simulink model "lab4_2"  (R2016b)
settings: Solver=VariableStepAuto  StartTime=0.0  StopTime=totaltime  RelTol=1e-3
undefined symbols (not defined in the file or in its folder): h
libraries: xbsIndex_r4 x1157
(part 1 of 4)
settings Model: Creator=rm101  LastModifiedBy=rm101

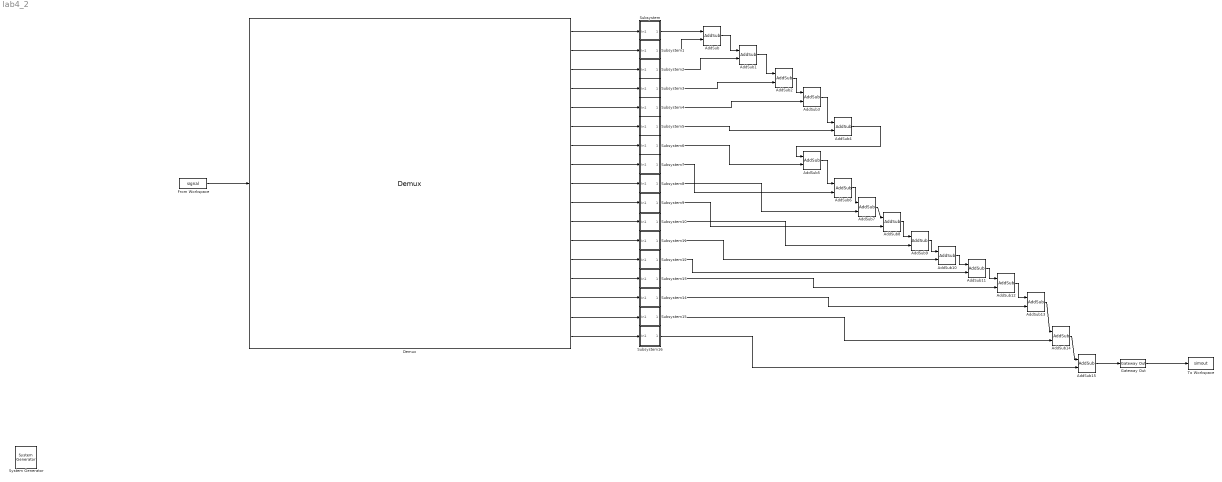
== system lab4_2 ==
  " System Generator" : xbsIndex_r4/ System Generator  Tag=genX  xilinxfamily=zynq  part=xc7z020  speed=-1  package=clg484  synthesis_tool=Vivado  clock_wrapper=Clock Enables  directory=C:/Users/rm101/lab4  proj_type=Vivado  Synth_file=Vivado Synthesis Defaults  Impl_file=Vivado Implementation Defaults  testbench=off  simulink_period=st  sysclk_period=10  dcm_input_clock_period=10  incr_netlist=off  trim_vbits=Everywhere in SubSystem  dbl_ovrd=According to Block Masks  core_generation=According to Block Masks  run_coregen=off  deprecated_control=off  eval_field=0  block_type=sysgen
  AddSub{,1..15} (16 alike) : xbsIndex_r4/AddSub  mode=Addition  use_carryin=off  use_carryout=off  en=off  latency=0  precision=Full  arith_type=Unsigned  n_bits=16  bin_pt=14  quantization=Truncate  overflow=Wrap  use_behavioral_HDL=off  hw_selection=Fabric  pipelined=off  dbl_ovrd=off  block_type=addsub
  Demux : Demux  Outputs=17
  From Workspace : FromWorkspace  VariableName=signal  SampleTime=0
  Gateway Out : xbsIndex_r4/Gateway Out  inherit_from_input=off  hdl_port=on  rows=1  columns=1  UseAsDAC=off  DACChannel='1'  interface=None  automatic_assignment=on  address_offset=hex2dec('00')  intf_name=''  intf_description=''  timing_constraint=None  locs_specified=off  LOCs={}  io_standard={}  block_type=gatewayout
  Subsystem : Subsystem
  Subsystem1 : Subsystem
  Subsystem10 : Subsystem
  Subsystem11 : Subsystem
  Subsystem12 : Subsystem
  Subsystem13 : Subsystem
  Subsystem14 : Subsystem
  Subsystem15 : Subsystem
  Subsystem16 : Subsystem
  Subsystem2 : Subsystem
  Subsystem3 : Subsystem
  Subsystem4 : Subsystem
  Subsystem5 : Subsystem
  Subsystem6 : Subsystem
  Subsystem7 : Subsystem
  Subsystem8 : Subsystem
  Subsystem9 : Subsystem
  To Workspace : ToWorkspace  VariableName=simout  SaveFormat=Timeseries  SampleTime=-1
  wires:
  From Workspace/1 -> Demux/1
  Demux/1 -> Subsystem/1(In1)
  Demux/2 -> Subsystem1/1(In1)
  Demux/3 -> Subsystem2/1(In1)
  Demux/4 -> Subsystem3/1(In1)
  Demux/5 -> Subsystem4/1(In1)
  Demux/6 -> Subsystem5/1(In1)
  Demux/7 -> Subsystem6/1(In1)
  Demux/8 -> Subsystem7/1(In1)
  Demux/9 -> Subsystem8/1(In1)
  Demux/10 -> Subsystem9/1(In1)
  Demux/11 -> Subsystem10/1(In1)
  Demux/12 -> Subsystem11/1(In1)
  Demux/13 -> Subsystem12/1(In1)
  Demux/14 -> Subsystem13/1(In1)
  Demux/15 -> Subsystem14/1(In1)
  Demux/16 -> Subsystem15/1(In1)
  Demux/17 -> Subsystem16/1(In1)
  Subsystem/1(Out1) -> AddSub/1
  Subsystem1/1(Out1) -> AddSub/2
  AddSub/1 -> AddSub1/1
  Subsystem2/1(Out1) -> AddSub1/2
  AddSub1/1 -> AddSub2/1
  Subsystem3/1(Out1) -> AddSub2/2
  AddSub2/1 -> AddSub3/1
  Subsystem4/1(Out1) -> AddSub3/2
  AddSub3/1 -> AddSub4/1
  Subsystem5/1(Out1) -> AddSub4/2
  Subsystem6/1(Out1) -> AddSub5/2
  Subsystem7/1(Out1) -> AddSub6/2
  AddSub5/1 -> AddSub6/1
  AddSub6/1 -> AddSub7/1
  AddSub7/1 -> AddSub8/1
  AddSub8/1 -> AddSub9/1
  AddSub9/1 -> AddSub10/1
  AddSub10/1 -> AddSub11/1
  AddSub11/1 -> AddSub12/1
  AddSub12/1 -> AddSub13/1
  AddSub13/1 -> AddSub14/1
  AddSub4/1 -> AddSub5/1
  Gateway Out/1 -> To Workspace/1
  Subsystem8/1(Out1) -> AddSub7/2
  Subsystem9/1(Out1) -> AddSub8/2
  Subsystem10/1(Out1) -> AddSub9/2
  Subsystem11/1(Out1) -> AddSub10/2
  Subsystem12/1(Out1) -> AddSub11/2
  Subsystem13/1(Out1) -> AddSub12/2
  Subsystem14/1(Out1) -> AddSub13/2
  Subsystem15/1(Out1) -> AddSub14/2
  AddSub15/1 -> Gateway Out/1
  AddSub14/1 -> AddSub15/1
  Subsystem16/1(Out1) -> AddSub15/2

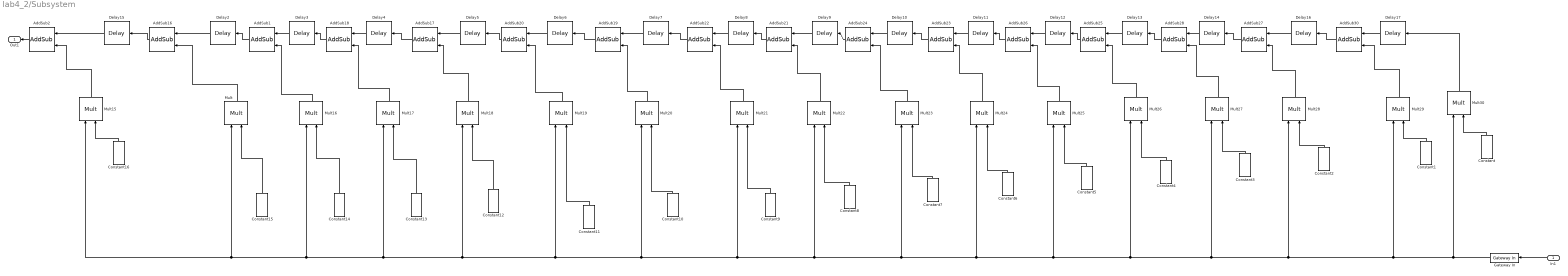
== system lab4_2/Subsystem ==
  In1 : Inport
  AddSub{1..2,16..28,30} (16 alike) : xbsIndex_r4/AddSub  mode=Addition  use_carryin=off  use_carryout=off  en=off  latency=0  precision=User Defined  arith_type="Signed  (2's comp)"  n_bits=W  bin_pt=B  quantization=Truncate  overflow=Wrap  use_behavioral_HDL=off  hw_selection=Fabric  pipelined=off  dbl_ovrd=off  block_type=addsub
  Constant : xbsIndex_r4/Constant  const=h(1,17)  gui_display_data_type=Fixed-point  arith_type=Signed (2's comp)  n_bits=W  bin_pt=B  preci_type=Single  exp_width=8  frac_width=24  explicit_period=off  period=1  equ=P=C  opselect=C  inp2=PCIN>>17  opr=+  inp1=P  carry=CIN  dbl_ovrd=off  block_type=constant
  Constant1 : xbsIndex_r4/Constant  const=h(2,17)  gui_display_data_type=Fixed-point  arith_type=Signed (2's comp)  n_bits=W  bin_pt=B  preci_type=Single  exp_width=8  frac_width=24  explicit_period=off  period=1  equ=P=C  opselect=C  inp2=PCIN>>17  opr=+  inp1=P  carry=CIN  dbl_ovrd=off  block_type=constant
  Constant10 : xbsIndex_r4/Constant  const=h(11,17)  gui_display_data_type=Fixed-point  arith_type=Signed (2's comp)  n_bits=W  bin_pt=B  preci_type=Single  exp_width=8  frac_width=24  explicit_period=off  period=1  equ=P=C  opselect=C  inp2=PCIN>>17  opr=+  inp1=P  carry=CIN  dbl_ovrd=off  block_type=constant
  Constant11 : xbsIndex_r4/Constant  const=h(12,17)  gui_display_data_type=Fixed-point  arith_type=Signed (2's comp)  n_bits=W  bin_pt=B  preci_type=Single  exp_width=8  frac_width=24  explicit_period=off  period=1  equ=P=C  opselect=C  inp2=PCIN>>17  opr=+  inp1=P  carry=CIN  dbl_ovrd=off  block_type=constant
  Constant12 : xbsIndex_r4/Constant  const=h(13,17)  gui_display_data_type=Fixed-point  arith_type=Signed (2's comp)  n_bits=W  bin_pt=B  preci_type=Single  exp_width=8  frac_width=24  explicit_period=off  period=1  equ=P=C  opselect=C  inp2=PCIN>>17  opr=+  inp1=P  carry=CIN  dbl_ovrd=off  block_type=constant
  Constant13 : xbsIndex_r4/Constant  const=h(14,17)  gui_display_data_type=Fixed-point  arith_type=Signed (2's comp)  n_bits=W  bin_pt=B  preci_type=Single  exp_width=8  frac_width=24  explicit_period=off  period=1  equ=P=C  opselect=C  inp2=PCIN>>17  opr=+  inp1=P  carry=CIN  dbl_ovrd=off  block_type=constant
  Constant14 : xbsIndex_r4/Constant  const=h(15,17)  gui_display_data_type=Fixed-point  arith_type=Signed (2's comp)  n_bits=W  bin_pt=B  preci_type=Single  exp_width=8  frac_width=24  explicit_period=off  period=1  equ=P=C  opselect=C  inp2=PCIN>>17  opr=+  inp1=P  carry=CIN  dbl_ovrd=off  block_type=constant
  Constant15 : xbsIndex_r4/Constant  const=h(16,17)  gui_display_data_type=Fixed-point  arith_type=Signed (2's comp)  n_bits=W  bin_pt=B  preci_type=Single  exp_width=8  frac_width=24  explicit_period=off  period=1  equ=P=C  opselect=C  inp2=PCIN>>17  opr=+  inp1=P  carry=CIN  dbl_ovrd=off  block_type=constant
  Constant16 : xbsIndex_r4/Constant  const=h(17,17)  gui_display_data_type=Fixed-point  arith_type=Signed (2's comp)  n_bits=W  bin_pt=B  preci_type=Single  exp_width=8  frac_width=24  explicit_period=off  period=1  equ=P=C  opselect=C  inp2=PCIN>>17  opr=+  inp1=P  carry=CIN  dbl_ovrd=off  block_type=constant
  Constant2 : xbsIndex_r4/Constant  const=h(3,17)  gui_display_data_type=Fixed-point  arith_type=Signed (2's comp)  n_bits=W  bin_pt=B  preci_type=Single  exp_width=8  frac_width=24  explicit_period=off  period=1  equ=P=C  opselect=C  inp2=PCIN>>17  opr=+  inp1=P  carry=CIN  dbl_ovrd=off  block_type=constant
  Constant3 : xbsIndex_r4/Constant  const=h(4,17)  gui_display_data_type=Fixed-point  arith_type=Signed (2's comp)  n_bits=W  bin_pt=B  preci_type=Single  exp_width=8  frac_width=24  explicit_period=off  period=1  equ=P=C  opselect=C  inp2=PCIN>>17  opr=+  inp1=P  carry=CIN  dbl_ovrd=off  block_type=constant
  Constant4 : xbsIndex_r4/Constant  const=h(5,17)  gui_display_data_type=Fixed-point  arith_type=Signed (2's comp)  n_bits=W  bin_pt=B  preci_type=Single  exp_width=8  frac_width=24  explicit_period=off  period=1  equ=P=C  opselect=C  inp2=PCIN>>17  opr=+  inp1=P  carry=CIN  dbl_ovrd=off  block_type=constant
  Constant5 : xbsIndex_r4/Constant  const=h(6,17)  gui_display_data_type=Fixed-point  arith_type=Signed (2's comp)  n_bits=W  bin_pt=B  preci_type=Single  exp_width=8  frac_width=24  explicit_period=off  period=1  equ=P=C  opselect=C  inp2=PCIN>>17  opr=+  inp1=P  carry=CIN  dbl_ovrd=off  block_type=constant
  Constant6 : xbsIndex_r4/Constant  const=h(7,17)  gui_display_data_type=Fixed-point  arith_type=Signed (2's comp)  n_bits=W  bin_pt=B  preci_type=Single  exp_width=8  frac_width=24  explicit_period=off  period=1  equ=P=C  opselect=C  inp2=PCIN>>17  opr=+  inp1=P  carry=CIN  dbl_ovrd=off  block_type=constant
  Constant7 : xbsIndex_r4/Constant  const=h(8,17)  gui_display_data_type=Fixed-point  arith_type=Signed (2's comp)  n_bits=W  bin_pt=B  preci_type=Single  exp_width=8  frac_width=24  explicit_period=off  period=1  equ=P=C  opselect=C  inp2=PCIN>>17  opr=+  inp1=P  carry=CIN  dbl_ovrd=off  block_type=constant
  Constant8 : xbsIndex_r4/Constant  const=h(9,17)  gui_display_data_type=Fixed-point  arith_type=Signed (2's comp)  n_bits=W  bin_pt=B  preci_type=Single  exp_width=8  frac_width=24  explicit_period=off  period=1  equ=P=C  opselect=C  inp2=PCIN>>17  opr=+  inp1=P  carry=CIN  dbl_ovrd=off  block_type=constant
  Constant9 : xbsIndex_r4/Constant  const=h(10,17)  gui_display_data_type=Fixed-point  arith_type=Signed (2's comp)  n_bits=W  bin_pt=B  preci_type=Single  exp_width=8  frac_width=24  explicit_period=off  period=1  equ=P=C  opselect=C  inp2=PCIN>>17  opr=+  inp1=P  carry=CIN  dbl_ovrd=off  block_type=constant
  Delay{2..17} (16 alike) : xbsIndex_r4/Delay  rst=off  infoeditControl=Selection of Reset will increase slice count due to use of real FFs and instead of SRLs  en=off  latency=1  reg_retiming=off  dbl_ovrd=off  block_type=delay
  Gateway In : xbsIndex_r4/Gateway In  gui_display_data_type=Fixed-point  arith_type="Signed  (2's comp)"  n_bits=W  bin_pt=B  preci_type=Single  exp_width=8  frac_width=24  rows=1  columns=1  quantization="Round  (unbiased: +/- Inf)"  overflow=Saturate  period=st  UseAsADC=off  ADCChannel='1'  interface=None  automatic_assignment=on  address_offset=hex2dec('00')  intf_name=''  intf_description=''  default_value=0  timing_constraint=None  locs_specified=off  LOCs={}  io_standard={}  inherit_from_input=off  hdl_port=on  dbl_ovrd=off  block_type=gatewayin
  Mult{,15..30} (17 alike) : xbsIndex_r4/Mult  precision=User Defined  arith_type="Signed  (2's comp)"  n_bits=W  bin_pt=B  quantization="Round  (unbiased: +/- Inf)"  overflow=Flag as error  en=off  latency=0  use_behavioral_HDL=off  opt=Speed  use_embedded=on  optimum_pipeline=off  pipeline=on  dbl_ovrd=off  use_rpm=on  placement_style=Triangular  block_type=mult
  Out1 : Outport
  wires:
  AddSub2/1 -> Out1/1
  Constant14/1 -> Mult16/2
  Mult/1 -> AddSub16/2
  Mult16/1 -> AddSub1/2
  AddSub16/1 -> Delay15/1
  Constant15/1 -> Mult/2
  AddSub1/1 -> Delay2/1
  Constant13/1 -> Mult17/2
  Mult17/1 -> AddSub18/2
  Constant12/1 -> Mult18/2
  AddSub17/1 -> Delay4/1
  AddSub18/1 -> Delay3/1
  Constant11/1 -> Mult19/2
  Mult19/1 -> AddSub20/2
  Constant10/1 -> Mult20/2
  Mult20/1 -> AddSub19/2
  AddSub19/1 -> Delay6/1
  AddSub20/1 -> Delay5/1
  Constant9/1 -> Mult21/2
  Mult21/1 -> AddSub22/2
  Constant8/1 -> Mult22/2
  AddSub21/1 -> Delay8/1
  AddSub22/1 -> Delay7/1
  Constant7/1 -> Mult23/2
  Mult23/1 -> AddSub24/2
  Constant6/1 -> Mult24/2
  AddSub23/1 -> Delay10/1
  Constant5/1 -> Mult25/2
  Mult25/1 -> AddSub26/2
  Constant4/1 -> Mult26/2
  Mult26/1 -> AddSub25/2
  AddSub25/1 -> Delay12/1
  AddSub26/1 -> Delay11/1
  Constant3/1 -> Mult27/2
  Mult27/1 -> AddSub28/2
  Constant2/1 -> Mult28/2
  AddSub27/1 -> Delay14/1
  AddSub28/1 -> Delay13/1
  Constant1/1 -> Mult29/2
  Mult29/1 -> AddSub30/2
  Constant/1 -> Mult30/2
  Mult30/1 -> Delay17/1
  AddSub30/1 -> Delay16/1
  AddSub24/1 -> Delay9/1
  Delay2/1 -> AddSub16/1
  Delay3/1 -> AddSub1/1
  Delay4/1 -> AddSub18/1
  Delay6/1 -> AddSub20/1
  Delay7/1 -> AddSub19/1
  Delay8/1 -> AddSub22/1
  Delay10/1 -> AddSub24/1
  Delay12/1 -> AddSub26/1
  Delay13/1 -> AddSub25/1
  Delay14/1 -> AddSub28/1
  Delay17/1 -> AddSub30/1
  Constant16/1 -> Mult15/2
  Mult15/1 -> AddSub2/2
  Delay15/1 -> AddSub2/1
  In1/1 -> Gateway In/1
  Delay5/1 -> AddSub17/1
  Mult18/1 -> AddSub17/2
  Delay9/1 -> AddSub21/1
  Mult22/1 -> AddSub21/2
  Delay11/1 -> AddSub23/1
  Mult24/1 -> AddSub23/2
  Delay16/1 -> AddSub27/1
  Mult28/1 -> AddSub27/2
  Gateway In/1 -> Mult30/1, Mult29/1, Mult28/1, Mult27/1, Mult26/1, Mult25/1, Mult24/1, Mult22/1, Mult21/1, Mult19/1, Mult17/1, Mult15/1, Mult/1, Mult16/1, Mult18/1, Mult20/1, Mult23/1

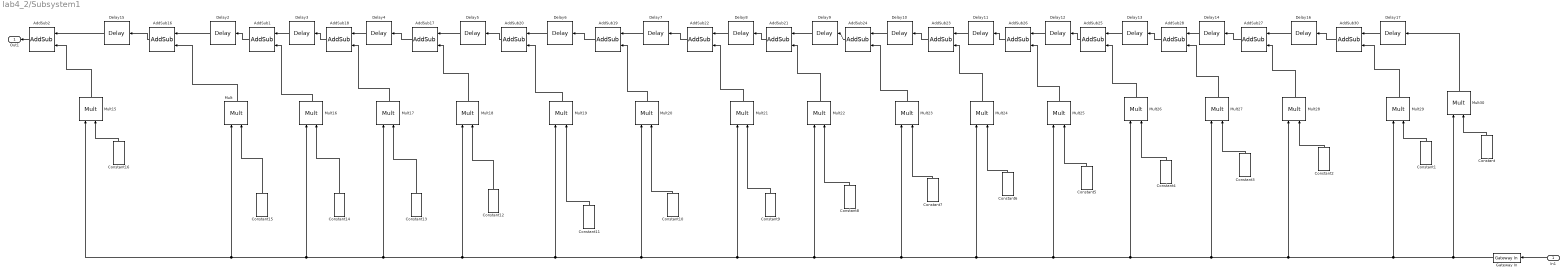
== system lab4_2/Subsystem1 ==
  In1 : Inport
  AddSub{1..2,16..28,30} (16 alike) : xbsIndex_r4/AddSub  mode=Addition  use_carryin=off  use_carryout=off  en=off  latency=0  precision=User Defined  arith_type="Signed  (2's comp)"  n_bits=W  bin_pt=B  quantization=Truncate  overflow=Wrap  use_behavioral_HDL=off  hw_selection=Fabric  pipelined=off  dbl_ovrd=off  block_type=addsub
  Constant : xbsIndex_r4/Constant  const=h(1,16)  gui_display_data_type=Fixed-point  arith_type=Signed (2's comp)  n_bits=W  bin_pt=B  preci_type=Single  exp_width=8  frac_width=24  explicit_period=off  period=1  equ=P=C  opselect=C  inp2=PCIN>>17  opr=+  inp1=P  carry=CIN  dbl_ovrd=off  block_type=constant
  Constant1 : xbsIndex_r4/Constant  const=h(2,16)  gui_display_data_type=Fixed-point  arith_type=Signed (2's comp)  n_bits=W  bin_pt=B  preci_type=Single  exp_width=8  frac_width=24  explicit_period=off  period=1  equ=P=C  opselect=C  inp2=PCIN>>17  opr=+  inp1=P  carry=CIN  dbl_ovrd=off  block_type=constant
  Constant10 : xbsIndex_r4/Constant  const=h(11,16)  gui_display_data_type=Fixed-point  arith_type=Signed (2's comp)  n_bits=W  bin_pt=B  preci_type=Single  exp_width=8  frac_width=24  explicit_period=off  period=1  equ=P=C  opselect=C  inp2=PCIN>>17  opr=+  inp1=P  carry=CIN  dbl_ovrd=off  block_type=constant
  Constant11 : xbsIndex_r4/Constant  const=h(12,16)  gui_display_data_type=Fixed-point  arith_type=Signed (2's comp)  n_bits=W  bin_pt=B  preci_type=Single  exp_width=8  frac_width=24  explicit_period=off  period=1  equ=P=C  opselect=C  inp2=PCIN>>17  opr=+  inp1=P  carry=CIN  dbl_ovrd=off  block_type=constant
  Constant12 : xbsIndex_r4/Constant  const=h(13,16)  gui_display_data_type=Fixed-point  arith_type=Signed (2's comp)  n_bits=W  bin_pt=B  preci_type=Single  exp_width=8  frac_width=24  explicit_period=off  period=1  equ=P=C  opselect=C  inp2=PCIN>>17  opr=+  inp1=P  carry=CIN  dbl_ovrd=off  block_type=constant
  Constant13 : xbsIndex_r4/Constant  const=h(14,16)  gui_display_data_type=Fixed-point  arith_type=Signed (2's comp)  n_bits=W  bin_pt=B  preci_type=Single  exp_width=8  frac_width=24  explicit_period=off  period=1  equ=P=C  opselect=C  inp2=PCIN>>17  opr=+  inp1=P  carry=CIN  dbl_ovrd=off  block_type=constant
  Constant14 : xbsIndex_r4/Constant  const=h(15,16)  gui_display_data_type=Fixed-point  arith_type=Signed (2's comp)  n_bits=W  bin_pt=B  preci_type=Single  exp_width=8  frac_width=24  explicit_period=off  period=1  equ=P=C  opselect=C  inp2=PCIN>>17  opr=+  inp1=P  carry=CIN  dbl_ovrd=off  block_type=constant
  Constant15 : xbsIndex_r4/Constant  const=h(16,16)  gui_display_data_type=Fixed-point  arith_type=Signed (2's comp)  n_bits=W  bin_pt=B  preci_type=Single  exp_width=8  frac_width=24  explicit_period=off  period=1  equ=P=C  opselect=C  inp2=PCIN>>17  opr=+  inp1=P  carry=CIN  dbl_ovrd=off  block_type=constant
  Constant16 : xbsIndex_r4/Constant  const=h(17,16)  gui_display_data_type=Fixed-point  arith_type=Signed (2's comp)  n_bits=W  bin_pt=B  preci_type=Single  exp_width=8  frac_width=24  explicit_period=off  period=1  equ=P=C  opselect=C  inp2=PCIN>>17  opr=+  inp1=P  carry=CIN  dbl_ovrd=off  block_type=constant
  Constant2 : xbsIndex_r4/Constant  const=h(3,16)  gui_display_data_type=Fixed-point  arith_type=Signed (2's comp)  n_bits=W  bin_pt=B  preci_type=Single  exp_width=8  frac_width=24  explicit_period=off  period=1  equ=P=C  opselect=C  inp2=PCIN>>17  opr=+  inp1=P  carry=CIN  dbl_ovrd=off  block_type=constant
  Constant3 : xbsIndex_r4/Constant  const=h(4,16)  gui_display_data_type=Fixed-point  arith_type=Signed (2's comp)  n_bits=W  bin_pt=B  preci_type=Single  exp_width=8  frac_width=24  explicit_period=off  period=1  equ=P=C  opselect=C  inp2=PCIN>>17  opr=+  inp1=P  carry=CIN  dbl_ovrd=off  block_type=constant
  Constant4 : xbsIndex_r4/Constant  const=h(5,16)  gui_display_data_type=Fixed-point  arith_type=Signed (2's comp)  n_bits=W  bin_pt=B  preci_type=Single  exp_width=8  frac_width=24  explicit_period=off  period=1  equ=P=C  opselect=C  inp2=PCIN>>17  opr=+  inp1=P  carry=CIN  dbl_ovrd=off  block_type=constant
  Constant5 : xbsIndex_r4/Constant  const=h(6,16)  gui_display_data_type=Fixed-point  arith_type=Signed (2's comp)  n_bits=W  bin_pt=B  preci_type=Single  exp_width=8  frac_width=24  explicit_period=off  period=1  equ=P=C  opselect=C  inp2=PCIN>>17  opr=+  inp1=P  carry=CIN  dbl_ovrd=off  block_type=constant
  Constant6 : xbsIndex_r4/Constant  const=h(7,16)  gui_display_data_type=Fixed-point  arith_type=Signed (2's comp)  n_bits=W  bin_pt=B  preci_type=Single  exp_width=8  frac_width=24  explicit_period=off  period=1  equ=P=C  opselect=C  inp2=PCIN>>17  opr=+  inp1=P  carry=CIN  dbl_ovrd=off  block_type=constant
  Constant7 : xbsIndex_r4/Constant  const=h(8,16)  gui_display_data_type=Fixed-point  arith_type=Signed (2's comp)  n_bits=W  bin_pt=B  preci_type=Single  exp_width=8  frac_width=24  explicit_period=off  period=1  equ=P=C  opselect=C  inp2=PCIN>>17  opr=+  inp1=P  carry=CIN  dbl_ovrd=off  block_type=constant
  Constant8 : xbsIndex_r4/Constant  const=h(9,16)  gui_display_data_type=Fixed-point  arith_type=Signed (2's comp)  n_bits=W  bin_pt=B  preci_type=Single  exp_width=8  frac_width=24  explicit_period=off  period=1  equ=P=C  opselect=C  inp2=PCIN>>17  opr=+  inp1=P  carry=CIN  dbl_ovrd=off  block_type=constant
  Constant9 : xbsIndex_r4/Constant  const=h(10,16)  gui_display_data_type=Fixed-point  arith_type=Signed (2's comp)  n_bits=W  bin_pt=B  preci_type=Single  exp_width=8  frac_width=24  explicit_period=off  period=1  equ=P=C  opselect=C  inp2=PCIN>>17  opr=+  inp1=P  carry=CIN  dbl_ovrd=off  block_type=constant
  Delay{2..17} (16 alike) : xbsIndex_r4/Delay  rst=off  infoeditControl=Selection of Reset will increase slice count due to use of real FFs and instead of SRLs  en=off  latency=1  reg_retiming=off  dbl_ovrd=off  block_type=delay
  Gateway In : xbsIndex_r4/Gateway In  gui_display_data_type=Fixed-point  arith_type="Signed  (2's comp)"  n_bits=W  bin_pt=B  preci_type=Single  exp_width=8  frac_width=24  rows=1  columns=1  quantization="Round  (unbiased: +/- Inf)"  overflow=Saturate  period=st  UseAsADC=off  ADCChannel='1'  interface=None  automatic_assignment=on  address_offset=hex2dec('00')  intf_name=''  intf_description=''  default_value=0  timing_constraint=None  locs_specified=off  LOCs={}  io_standard={}  inherit_from_input=off  hdl_port=on  dbl_ovrd=off  block_type=gatewayin
  Mult{,15..30} (17 alike) : xbsIndex_r4/Mult  precision=User Defined  arith_type="Signed  (2's comp)"  n_bits=W  bin_pt=B  quantization="Round  (unbiased: +/- Inf)"  overflow=Flag as error  en=off  latency=0  use_behavioral_HDL=off  opt=Speed  use_embedded=on  optimum_pipeline=off  pipeline=on  dbl_ovrd=off  use_rpm=on  placement_style=Triangular  block_type=mult
  Out1 : Outport
  wires:
  AddSub2/1 -> Out1/1
  Constant14/1 -> Mult16/2
  Mult/1 -> AddSub16/2
  Mult16/1 -> AddSub1/2
  AddSub16/1 -> Delay15/1
  Constant15/1 -> Mult/2
  AddSub1/1 -> Delay2/1
  Constant13/1 -> Mult17/2
  Mult17/1 -> AddSub18/2
  Constant12/1 -> Mult18/2
  AddSub17/1 -> Delay4/1
  AddSub18/1 -> Delay3/1
  Constant11/1 -> Mult19/2
  Mult19/1 -> AddSub20/2
  Constant10/1 -> Mult20/2
  Mult20/1 -> AddSub19/2
  AddSub19/1 -> Delay6/1
  AddSub20/1 -> Delay5/1
  Constant9/1 -> Mult21/2
  Mult21/1 -> AddSub22/2
  Constant8/1 -> Mult22/2
  AddSub21/1 -> Delay8/1
  AddSub22/1 -> Delay7/1
  Constant7/1 -> Mult23/2
  Mult23/1 -> AddSub24/2
  Constant6/1 -> Mult24/2
  AddSub23/1 -> Delay10/1
  Constant5/1 -> Mult25/2
  Mult25/1 -> AddSub26/2
  Constant4/1 -> Mult26/2
  Mult26/1 -> AddSub25/2
  AddSub25/1 -> Delay12/1
  AddSub26/1 -> Delay11/1
  Constant3/1 -> Mult27/2
  Mult27/1 -> AddSub28/2
  Constant2/1 -> Mult28/2
  AddSub27/1 -> Delay14/1
  AddSub28/1 -> Delay13/1
  Constant1/1 -> Mult29/2
  Mult29/1 -> AddSub30/2
  Constant/1 -> Mult30/2
  Mult30/1 -> Delay17/1
  AddSub30/1 -> Delay16/1
  AddSub24/1 -> Delay9/1
  Delay2/1 -> AddSub16/1
  Delay3/1 -> AddSub1/1
  Delay4/1 -> AddSub18/1
  Delay6/1 -> AddSub20/1
  Delay7/1 -> AddSub19/1
  Delay8/1 -> AddSub22/1
  Delay10/1 -> AddSub24/1
  Delay12/1 -> AddSub26/1
  Delay13/1 -> AddSub25/1
  Delay14/1 -> AddSub28/1
  Delay17/1 -> AddSub30/1
  Constant16/1 -> Mult15/2
  Mult15/1 -> AddSub2/2
  Delay15/1 -> AddSub2/1
  In1/1 -> Gateway In/1
  Delay5/1 -> AddSub17/1
  Mult18/1 -> AddSub17/2
  Delay9/1 -> AddSub21/1
  Mult22/1 -> AddSub21/2
  Delay11/1 -> AddSub23/1
  Mult24/1 -> AddSub23/2
  Delay16/1 -> AddSub27/1
  Mult28/1 -> AddSub27/2
  Gateway In/1 -> Mult30/1, Mult29/1, Mult28/1, Mult27/1, Mult26/1, Mult25/1, Mult24/1, Mult22/1, Mult21/1, Mult19/1, Mult17/1, Mult15/1, Mult/1, Mult16/1, Mult18/1, Mult20/1, Mult23/1

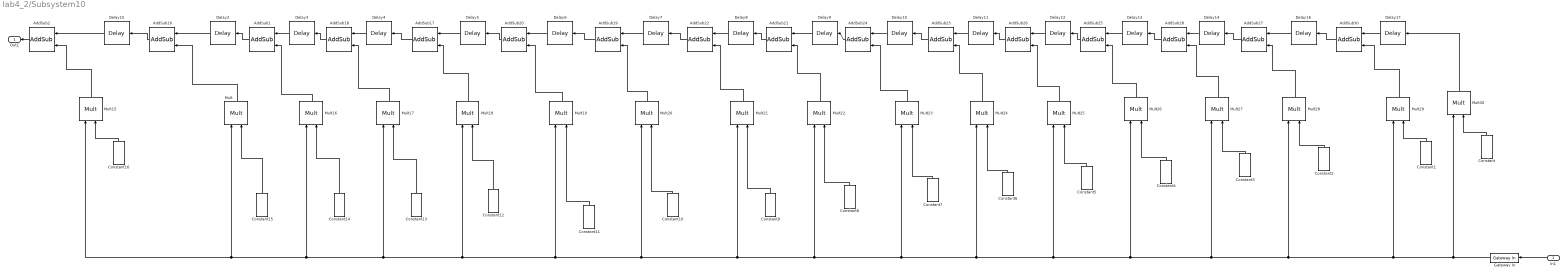
== system lab4_2/Subsystem10 ==
  In1 : Inport
  AddSub{1..2,16..28,30} (16 alike) : xbsIndex_r4/AddSub  mode=Addition  use_carryin=off  use_carryout=off  en=off  latency=0  precision=User Defined  arith_type="Signed  (2's comp)"  n_bits=W  bin_pt=B  quantization=Truncate  overflow=Wrap  use_behavioral_HDL=off  hw_selection=Fabric  pipelined=off  dbl_ovrd=off  block_type=addsub
  Constant : xbsIndex_r4/Constant  const=h(1,7)  gui_display_data_type=Fixed-point  arith_type=Signed (2's comp)  n_bits=W  bin_pt=B  preci_type=Single  exp_width=8  frac_width=24  explicit_period=off  period=1  equ=P=C  opselect=C  inp2=PCIN>>17  opr=+  inp1=P  carry=CIN  dbl_ovrd=off  block_type=constant
  Constant1 : xbsIndex_r4/Constant  const=h(2,7)  gui_display_data_type=Fixed-point  arith_type=Signed (2's comp)  n_bits=W  bin_pt=B  preci_type=Single  exp_width=8  frac_width=24  explicit_period=off  period=1  equ=P=C  opselect=C  inp2=PCIN>>17  opr=+  inp1=P  carry=CIN  dbl_ovrd=off  block_type=constant
  Constant10 : xbsIndex_r4/Constant  const=h(11,7)  gui_display_data_type=Fixed-point  arith_type=Signed (2's comp)  n_bits=W  bin_pt=B  preci_type=Single  exp_width=8  frac_width=24  explicit_period=off  period=1  equ=P=C  opselect=C  inp2=PCIN>>17  opr=+  inp1=P  carry=CIN  dbl_ovrd=off  block_type=constant
  Constant11 : xbsIndex_r4/Constant  const=h(12,7)  gui_display_data_type=Fixed-point  arith_type=Signed (2's comp)  n_bits=W  bin_pt=B  preci_type=Single  exp_width=8  frac_width=24  explicit_period=off  period=1  equ=P=C  opselect=C  inp2=PCIN>>17  opr=+  inp1=P  carry=CIN  dbl_ovrd=off  block_type=constant
  Constant12 : xbsIndex_r4/Constant  const=h(13,7)  gui_display_data_type=Fixed-point  arith_type=Signed (2's comp)  n_bits=W  bin_pt=B  preci_type=Single  exp_width=8  frac_width=24  explicit_period=off  period=1  equ=P=C  opselect=C  inp2=PCIN>>17  opr=+  inp1=P  carry=CIN  dbl_ovrd=off  block_type=constant
  Constant13 : xbsIndex_r4/Constant  const=h(14,7)  gui_display_data_type=Fixed-point  arith_type=Signed (2's comp)  n_bits=W  bin_pt=B  preci_type=Single  exp_width=8  frac_width=24  explicit_period=off  period=1  equ=P=C  opselect=C  inp2=PCIN>>17  opr=+  inp1=P  carry=CIN  dbl_ovrd=off  block_type=constant
  Constant14 : xbsIndex_r4/Constant  const=h(15,7)  gui_display_data_type=Fixed-point  arith_type=Signed (2's comp)  n_bits=W  bin_pt=B  preci_type=Single  exp_width=8  frac_width=24  explicit_period=off  period=1  equ=P=C  opselect=C  inp2=PCIN>>17  opr=+  inp1=P  carry=CIN  dbl_ovrd=off  block_type=constant
  Constant15 : xbsIndex_r4/Constant  const=h(16,7)  gui_display_data_type=Fixed-point  arith_type=Signed (2's comp)  n_bits=W  bin_pt=B  preci_type=Single  exp_width=8  frac_width=24  explicit_period=off  period=1  equ=P=C  opselect=C  inp2=PCIN>>17  opr=+  inp1=P  carry=CIN  dbl_ovrd=off  block_type=constant
  Constant16 : xbsIndex_r4/Constant  const=h(17,7)  gui_display_data_type=Fixed-point  arith_type=Signed (2's comp)  n_bits=W  bin_pt=B  preci_type=Single  exp_width=8  frac_width=24  explicit_period=off  period=1  equ=P=C  opselect=C  inp2=PCIN>>17  opr=+  inp1=P  carry=CIN  dbl_ovrd=off  block_type=constant
  Constant2 : xbsIndex_r4/Constant  const=h(3,7)  gui_display_data_type=Fixed-point  arith_type=Signed (2's comp)  n_bits=W  bin_pt=B  preci_type=Single  exp_width=8  frac_width=24  explicit_period=off  period=1  equ=P=C  opselect=C  inp2=PCIN>>17  opr=+  inp1=P  carry=CIN  dbl_ovrd=off  block_type=constant
  Constant3 : xbsIndex_r4/Constant  const=h(4,7)  gui_display_data_type=Fixed-point  arith_type=Signed (2's comp)  n_bits=W  bin_pt=B  preci_type=Single  exp_width=8  frac_width=24  explicit_period=off  period=1  equ=P=C  opselect=C  inp2=PCIN>>17  opr=+  inp1=P  carry=CIN  dbl_ovrd=off  block_type=constant
  Constant4 : xbsIndex_r4/Constant  const=h(5,7)  gui_display_data_type=Fixed-point  arith_type=Signed (2's comp)  n_bits=W  bin_pt=B  preci_type=Single  exp_width=8  frac_width=24  explicit_period=off  period=1  equ=P=C  opselect=C  inp2=PCIN>>17  opr=+  inp1=P  carry=CIN  dbl_ovrd=off  block_type=constant
  Constant5 : xbsIndex_r4/Constant  const=h(6,7)  gui_display_data_type=Fixed-point  arith_type=Signed (2's comp)  n_bits=W  bin_pt=B  preci_type=Single  exp_width=8  frac_width=24  explicit_period=off  period=1  equ=P=C  opselect=C  inp2=PCIN>>17  opr=+  inp1=P  carry=CIN  dbl_ovrd=off  block_type=constant
  Constant6 : xbsIndex_r4/Constant  const=h(7,7)  gui_display_data_type=Fixed-point  arith_type=Signed (2's comp)  n_bits=W  bin_pt=B  preci_type=Single  exp_width=8  frac_width=24  explicit_period=off  period=1  equ=P=C  opselect=C  inp2=PCIN>>17  opr=+  inp1=P  carry=CIN  dbl_ovrd=off  block_type=constant
  Constant7 : xbsIndex_r4/Constant  const=h(8,7)  gui_display_data_type=Fixed-point  arith_type=Signed (2's comp)  n_bits=W  bin_pt=B  preci_type=Single  exp_width=8  frac_width=24  explicit_period=off  period=1  equ=P=C  opselect=C  inp2=PCIN>>17  opr=+  inp1=P  carry=CIN  dbl_ovrd=off  block_type=constant
  Constant8 : xbsIndex_r4/Constant  const=h(9,7)  gui_display_data_type=Fixed-point  arith_type=Signed (2's comp)  n_bits=W  bin_pt=B  preci_type=Single  exp_width=8  frac_width=24  explicit_period=off  period=1  equ=P=C  opselect=C  inp2=PCIN>>17  opr=+  inp1=P  carry=CIN  dbl_ovrd=off  block_type=constant
  Constant9 : xbsIndex_r4/Constant  const=h(10,7)  gui_display_data_type=Fixed-point  arith_type=Signed (2's comp)  n_bits=W  bin_pt=B  preci_type=Single  exp_width=8  frac_width=24  explicit_period=off  period=1  equ=P=C  opselect=C  inp2=PCIN>>17  opr=+  inp1=P  carry=CIN  dbl_ovrd=off  block_type=constant
  Delay{2..17} (16 alike) : xbsIndex_r4/Delay  rst=off  infoeditControl=Selection of Reset will increase slice count due to use of real FFs and instead of SRLs  en=off  latency=1  reg_retiming=off  dbl_ovrd=off  block_type=delay
  Gateway In : xbsIndex_r4/Gateway In  gui_display_data_type=Fixed-point  arith_type="Signed  (2's comp)"  n_bits=W  bin_pt=B  preci_type=Single  exp_width=8  frac_width=24  rows=1  columns=1  quantization="Round  (unbiased: +/- Inf)"  overflow=Saturate  period=st  UseAsADC=off  ADCChannel='1'  interface=None  automatic_assignment=on  address_offset=hex2dec('00')  intf_name=''  intf_description=''  default_value=0  timing_constraint=None  locs_specified=off  LOCs={}  io_standard={}  inherit_from_input=off  hdl_port=on  dbl_ovrd=off  block_type=gatewayin
  Mult{,15..30} (17 alike) : xbsIndex_r4/Mult  precision=User Defined  arith_type="Signed  (2's comp)"  n_bits=W  bin_pt=B  quantization="Round  (unbiased: +/- Inf)"  overflow=Flag as error  en=off  latency=0  use_behavioral_HDL=off  opt=Speed  use_embedded=on  optimum_pipeline=off  pipeline=on  dbl_ovrd=off  use_rpm=on  placement_style=Triangular  block_type=mult
  Out1 : Outport
  wires:
  AddSub2/1 -> Out1/1
  Constant14/1 -> Mult16/2
  Mult/1 -> AddSub16/2
  Mult16/1 -> AddSub1/2
  AddSub16/1 -> Delay15/1
  Constant15/1 -> Mult/2
  AddSub1/1 -> Delay2/1
  Constant13/1 -> Mult17/2
  Mult17/1 -> AddSub18/2
  Constant12/1 -> Mult18/2
  AddSub17/1 -> Delay4/1
  AddSub18/1 -> Delay3/1
  Constant11/1 -> Mult19/2
  Mult19/1 -> AddSub20/2
  Constant10/1 -> Mult20/2
  Mult20/1 -> AddSub19/2
  AddSub19/1 -> Delay6/1
  AddSub20/1 -> Delay5/1
  Constant9/1 -> Mult21/2
  Mult21/1 -> AddSub22/2
  Constant8/1 -> Mult22/2
  AddSub21/1 -> Delay8/1
  AddSub22/1 -> Delay7/1
  Constant7/1 -> Mult23/2
  Mult23/1 -> AddSub24/2
  Constant6/1 -> Mult24/2
  AddSub23/1 -> Delay10/1
  Constant5/1 -> Mult25/2
  Mult25/1 -> AddSub26/2
  Constant4/1 -> Mult26/2
  Mult26/1 -> AddSub25/2
  AddSub25/1 -> Delay12/1
  AddSub26/1 -> Delay11/1
  Constant3/1 -> Mult27/2
  Mult27/1 -> AddSub28/2
  Constant2/1 -> Mult28/2
  AddSub27/1 -> Delay14/1
  AddSub28/1 -> Delay13/1
  Constant1/1 -> Mult29/2
  Mult29/1 -> AddSub30/2
  Constant/1 -> Mult30/2
  Mult30/1 -> Delay17/1
  AddSub30/1 -> Delay16/1
  AddSub24/1 -> Delay9/1
  Delay2/1 -> AddSub16/1
  Delay3/1 -> AddSub1/1
  Delay4/1 -> AddSub18/1
  Delay6/1 -> AddSub20/1
  Delay7/1 -> AddSub19/1
  Delay8/1 -> AddSub22/1
  Delay10/1 -> AddSub24/1
  Delay12/1 -> AddSub26/1
  Delay13/1 -> AddSub25/1
  Delay14/1 -> AddSub28/1
  Delay17/1 -> AddSub30/1
  Constant16/1 -> Mult15/2
  Mult15/1 -> AddSub2/2
  Delay15/1 -> AddSub2/1
  In1/1 -> Gateway In/1
  Delay5/1 -> AddSub17/1
  Mult18/1 -> AddSub17/2
  Delay9/1 -> AddSub21/1
  Mult22/1 -> AddSub21/2
  Delay11/1 -> AddSub23/1
  Mult24/1 -> AddSub23/2
  Delay16/1 -> AddSub27/1
  Mult28/1 -> AddSub27/2
  Gateway In/1 -> Mult30/1, Mult29/1, Mult28/1, Mult27/1, Mult26/1, Mult25/1, Mult24/1, Mult22/1, Mult21/1, Mult19/1, Mult17/1, Mult15/1, Mult/1, Mult16/1, Mult18/1, Mult20/1, Mult23/1

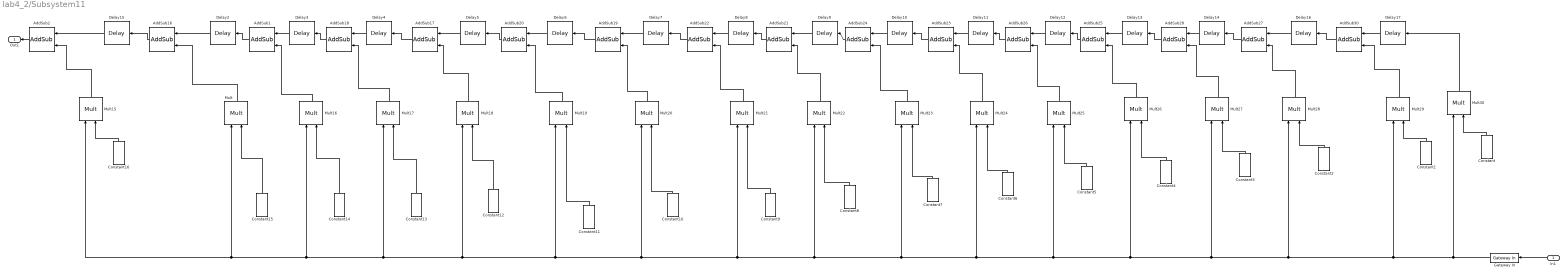
== system lab4_2/Subsystem11 ==
  In1 : Inport
  AddSub{1..2,16..28,30} (16 alike) : xbsIndex_r4/AddSub  mode=Addition  use_carryin=off  use_carryout=off  en=off  latency=0  precision=User Defined  arith_type="Signed  (2's comp)"  n_bits=W  bin_pt=B  quantization=Truncate  overflow=Wrap  use_behavioral_HDL=off  hw_selection=Fabric  pipelined=off  dbl_ovrd=off  block_type=addsub
  Constant : xbsIndex_r4/Constant  const=h(1,6)  gui_display_data_type=Fixed-point  arith_type=Signed (2's comp)  n_bits=W  bin_pt=B  preci_type=Single  exp_width=8  frac_width=24  explicit_period=off  period=1  equ=P=C  opselect=C  inp2=PCIN>>17  opr=+  inp1=P  carry=CIN  dbl_ovrd=off  block_type=constant
  Constant1 : xbsIndex_r4/Constant  const=h(2,6)  gui_display_data_type=Fixed-point  arith_type=Signed (2's comp)  n_bits=W  bin_pt=B  preci_type=Single  exp_width=8  frac_width=24  explicit_period=off  period=1  equ=P=C  opselect=C  inp2=PCIN>>17  opr=+  inp1=P  carry=CIN  dbl_ovrd=off  block_type=constant
  Constant10 : xbsIndex_r4/Constant  const=h(11,6)  gui_display_data_type=Fixed-point  arith_type=Signed (2's comp)  n_bits=W  bin_pt=B  preci_type=Single  exp_width=8  frac_width=24  explicit_period=off  period=1  equ=P=C  opselect=C  inp2=PCIN>>17  opr=+  inp1=P  carry=CIN  dbl_ovrd=off  block_type=constant
  Constant11 : xbsIndex_r4/Constant  const=h(12,6)  gui_display_data_type=Fixed-point  arith_type=Signed (2's comp)  n_bits=W  bin_pt=B  preci_type=Single  exp_width=8  frac_width=24  explicit_period=off  period=1  equ=P=C  opselect=C  inp2=PCIN>>17  opr=+  inp1=P  carry=CIN  dbl_ovrd=off  block_type=constant
  Constant12 : xbsIndex_r4/Constant  const=h(13,6)  gui_display_data_type=Fixed-point  arith_type=Signed (2's comp)  n_bits=W  bin_pt=B  preci_type=Single  exp_width=8  frac_width=24  explicit_period=off  period=1  equ=P=C  opselect=C  inp2=PCIN>>17  opr=+  inp1=P  carry=CIN  dbl_ovrd=off  block_type=constant
  Constant13 : xbsIndex_r4/Constant  const=h(14,6)  gui_display_data_type=Fixed-point  arith_type=Signed (2's comp)  n_bits=W  bin_pt=B  preci_type=Single  exp_width=8  frac_width=24  explicit_period=off  period=1  equ=P=C  opselect=C  inp2=PCIN>>17  opr=+  inp1=P  carry=CIN  dbl_ovrd=off  block_type=constant
  Constant14 : xbsIndex_r4/Constant  const=h(15,6)  gui_display_data_type=Fixed-point  arith_type=Signed (2's comp)  n_bits=W  bin_pt=B  preci_type=Single  exp_width=8  frac_width=24  explicit_period=off  period=1  equ=P=C  opselect=C  inp2=PCIN>>17  opr=+  inp1=P  carry=CIN  dbl_ovrd=off  block_type=constant
  Constant15 : xbsIndex_r4/Constant  const=h(16,6)  gui_display_data_type=Fixed-point  arith_type=Signed (2's comp)  n_bits=W  bin_pt=B  preci_type=Single  exp_width=8  frac_width=24  explicit_period=off  period=1  equ=P=C  opselect=C  inp2=PCIN>>17  opr=+  inp1=P  carry=CIN  dbl_ovrd=off  block_type=constant
  Constant16 : xbsIndex_r4/Constant  const=h(17,6)  gui_display_data_type=Fixed-point  arith_type=Signed (2's comp)  n_bits=W  bin_pt=B  preci_type=Single  exp_width=8  frac_width=24  explicit_period=off  period=1  equ=P=C  opselect=C  inp2=PCIN>>17  opr=+  inp1=P  carry=CIN  dbl_ovrd=off  block_type=constant
  Constant2 : xbsIndex_r4/Constant  const=h(3,6)  gui_display_data_type=Fixed-point  arith_type=Signed (2's comp)  n_bits=W  bin_pt=B  preci_type=Single  exp_width=8  frac_width=24  explicit_period=off  period=1  equ=P=C  opselect=C  inp2=PCIN>>17  opr=+  inp1=P  carry=CIN  dbl_ovrd=off  block_type=constant
  Constant3 : xbsIndex_r4/Constant  const=h(4,6)  gui_display_data_type=Fixed-point  arith_type=Signed (2's comp)  n_bits=W  bin_pt=B  preci_type=Single  exp_width=8  frac_width=24  explicit_period=off  period=1  equ=P=C  opselect=C  inp2=PCIN>>17  opr=+  inp1=P  carry=CIN  dbl_ovrd=off  block_type=constant
  Constant4 : xbsIndex_r4/Constant  const=h(5,6)  gui_display_data_type=Fixed-point  arith_type=Signed (2's comp)  n_bits=W  bin_pt=B  preci_type=Single  exp_width=8  frac_width=24  explicit_period=off  period=1  equ=P=C  opselect=C  inp2=PCIN>>17  opr=+  inp1=P  carry=CIN  dbl_ovrd=off  block_type=constant
  Constant5 : xbsIndex_r4/Constant  const=h(6,6)  gui_display_data_type=Fixed-point  arith_type=Signed (2's comp)  n_bits=W  bin_pt=B  preci_type=Single  exp_width=8  frac_width=24  explicit_period=off  period=1  equ=P=C  opselect=C  inp2=PCIN>>17  opr=+  inp1=P  carry=CIN  dbl_ovrd=off  block_type=constant
  Constant6 : xbsIndex_r4/Constant  const=h(7,6)  gui_display_data_type=Fixed-point  arith_type=Signed (2's comp)  n_bits=W  bin_pt=B  preci_type=Single  exp_width=8  frac_width=24  explicit_period=off  period=1  equ=P=C  opselect=C  inp2=PCIN>>17  opr=+  inp1=P  carry=CIN  dbl_ovrd=off  block_type=constant
  Constant7 : xbsIndex_r4/Constant  const=h(8,6)  gui_display_data_type=Fixed-point  arith_type=Signed (2's comp)  n_bits=W  bin_pt=B  preci_type=Single  exp_width=8  frac_width=24  explicit_period=off  period=1  equ=P=C  opselect=C  inp2=PCIN>>17  opr=+  inp1=P  carry=CIN  dbl_ovrd=off  block_type=constant
  Constant8 : xbsIndex_r4/Constant  const=h(9,6)  gui_display_data_type=Fixed-point  arith_type=Signed (2's comp)  n_bits=W  bin_pt=B  preci_type=Single  exp_width=8  frac_width=24  explicit_period=off  period=1  equ=P=C  opselect=C  inp2=PCIN>>17  opr=+  inp1=P  carry=CIN  dbl_ovrd=off  block_type=constant
  Constant9 : xbsIndex_r4/Constant  const=h(10,6)  gui_display_data_type=Fixed-point  arith_type=Signed (2's comp)  n_bits=W  bin_pt=B  preci_type=Single  exp_width=8  frac_width=24  explicit_period=off  period=1  equ=P=C  opselect=C  inp2=PCIN>>17  opr=+  inp1=P  carry=CIN  dbl_ovrd=off  block_type=constant
  Delay{2..17} (16 alike) : xbsIndex_r4/Delay  rst=off  infoeditControl=Selection of Reset will increase slice count due to use of real FFs and instead of SRLs  en=off  latency=1  reg_retiming=off  dbl_ovrd=off  block_type=delay
  Gateway In : xbsIndex_r4/Gateway In  gui_display_data_type=Fixed-point  arith_type="Signed  (2's comp)"  n_bits=W  bin_pt=B  preci_type=Single  exp_width=8  frac_width=24  rows=1  columns=1  quantization="Round  (unbiased: +/- Inf)"  overflow=Saturate  period=st  UseAsADC=off  ADCChannel='1'  interface=None  automatic_assignment=on  address_offset=hex2dec('00')  intf_name=''  intf_description=''  default_value=0  timing_constraint=None  locs_specified=off  LOCs={}  io_standard={}  inherit_from_input=off  hdl_port=on  dbl_ovrd=off  block_type=gatewayin
  Mult{,15..30} (17 alike) : xbsIndex_r4/Mult  precision=User Defined  arith_type="Signed  (2's comp)"  n_bits=W  bin_pt=B  quantization="Round  (unbiased: +/- Inf)"  overflow=Flag as error  en=off  latency=0  use_behavioral_HDL=off  opt=Speed  use_embedded=on  optimum_pipeline=off  pipeline=on  dbl_ovrd=off  use_rpm=on  placement_style=Triangular  block_type=mult
  Out1 : Outport
  wires:
  AddSub2/1 -> Out1/1
  Constant14/1 -> Mult16/2
  Mult/1 -> AddSub16/2
  Mult16/1 -> AddSub1/2
  AddSub16/1 -> Delay15/1
  Constant15/1 -> Mult/2
  AddSub1/1 -> Delay2/1
  Constant13/1 -> Mult17/2
  Mult17/1 -> AddSub18/2
  Constant12/1 -> Mult18/2
  AddSub17/1 -> Delay4/1
  AddSub18/1 -> Delay3/1
  Constant11/1 -> Mult19/2
  Mult19/1 -> AddSub20/2
  Constant10/1 -> Mult20/2
  Mult20/1 -> AddSub19/2
  AddSub19/1 -> Delay6/1
  AddSub20/1 -> Delay5/1
  Constant9/1 -> Mult21/2
  Mult21/1 -> AddSub22/2
  Constant8/1 -> Mult22/2
  AddSub21/1 -> Delay8/1
  AddSub22/1 -> Delay7/1
  Constant7/1 -> Mult23/2
  Mult23/1 -> AddSub24/2
  Constant6/1 -> Mult24/2
  AddSub23/1 -> Delay10/1
  Constant5/1 -> Mult25/2
  Mult25/1 -> AddSub26/2
  Constant4/1 -> Mult26/2
  Mult26/1 -> AddSub25/2
  AddSub25/1 -> Delay12/1
  AddSub26/1 -> Delay11/1
  Constant3/1 -> Mult27/2
  Mult27/1 -> AddSub28/2
  Constant2/1 -> Mult28/2
  AddSub27/1 -> Delay14/1
  AddSub28/1 -> Delay13/1
  Constant1/1 -> Mult29/2
  Mult29/1 -> AddSub30/2
  Constant/1 -> Mult30/2
  Mult30/1 -> Delay17/1
  AddSub30/1 -> Delay16/1
  AddSub24/1 -> Delay9/1
  Delay2/1 -> AddSub16/1
  Delay3/1 -> AddSub1/1
  Delay4/1 -> AddSub18/1
  Delay6/1 -> AddSub20/1
  Delay7/1 -> AddSub19/1
  Delay8/1 -> AddSub22/1
  Delay10/1 -> AddSub24/1
  Delay12/1 -> AddSub26/1
  Delay13/1 -> AddSub25/1
  Delay14/1 -> AddSub28/1
  Delay17/1 -> AddSub30/1
  Constant16/1 -> Mult15/2
  Mult15/1 -> AddSub2/2
  Delay15/1 -> AddSub2/1
  In1/1 -> Gateway In/1
  Delay5/1 -> AddSub17/1
  Mult18/1 -> AddSub17/2
  Delay9/1 -> AddSub21/1
  Mult22/1 -> AddSub21/2
  Delay11/1 -> AddSub23/1
  Mult24/1 -> AddSub23/2
  Delay16/1 -> AddSub27/1
  Mult28/1 -> AddSub27/2
  Gateway In/1 -> Mult30/1, Mult29/1, Mult28/1, Mult27/1, Mult26/1, Mult25/1, Mult24/1, Mult22/1, Mult21/1, Mult19/1, Mult17/1, Mult15/1, Mult/1, Mult16/1, Mult18/1, Mult20/1, Mult23/1

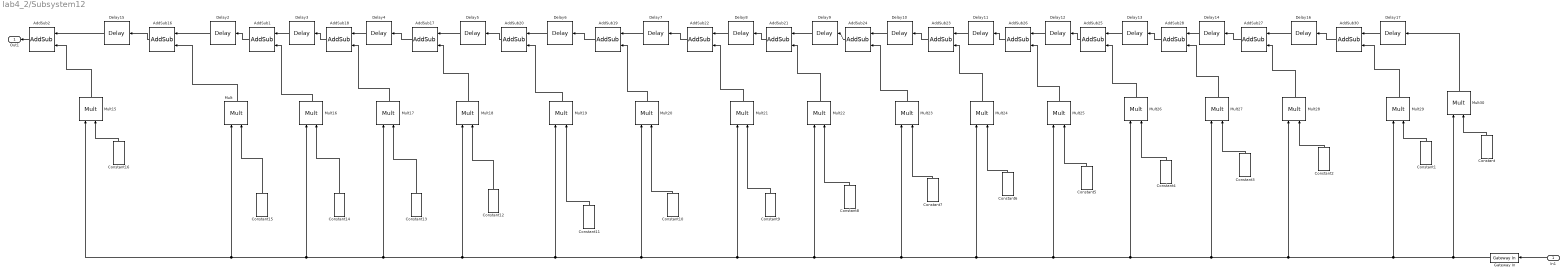
== system lab4_2/Subsystem12 ==
  In1 : Inport
  AddSub{1..2,16..28,30} (16 alike) : xbsIndex_r4/AddSub  mode=Addition  use_carryin=off  use_carryout=off  en=off  latency=0  precision=User Defined  arith_type="Signed  (2's comp)"  n_bits=W  bin_pt=B  quantization=Truncate  overflow=Wrap  use_behavioral_HDL=off  hw_selection=Fabric  pipelined=off  dbl_ovrd=off  block_type=addsub
  Constant : xbsIndex_r4/Constant  const=h(1,5)  gui_display_data_type=Fixed-point  arith_type=Signed (2's comp)  n_bits=W  bin_pt=B  preci_type=Single  exp_width=8  frac_width=24  explicit_period=off  period=1  equ=P=C  opselect=C  inp2=PCIN>>17  opr=+  inp1=P  carry=CIN  dbl_ovrd=off  block_type=constant
  Constant1 : xbsIndex_r4/Constant  const=h(2,5)  gui_display_data_type=Fixed-point  arith_type=Signed (2's comp)  n_bits=W  bin_pt=B  preci_type=Single  exp_width=8  frac_width=24  explicit_period=off  period=1  equ=P=C  opselect=C  inp2=PCIN>>17  opr=+  inp1=P  carry=CIN  dbl_ovrd=off  block_type=constant
  Constant10 : xbsIndex_r4/Constant  const=h(11,5)  gui_display_data_type=Fixed-point  arith_type=Signed (2's comp)  n_bits=W  bin_pt=B  preci_type=Single  exp_width=8  frac_width=24  explicit_period=off  period=1  equ=P=C  opselect=C  inp2=PCIN>>17  opr=+  inp1=P  carry=CIN  dbl_ovrd=off  block_type=constant
  Constant11 : xbsIndex_r4/Constant  const=h(12,5)  gui_display_data_type=Fixed-point  arith_type=Signed (2's comp)  n_bits=W  bin_pt=B  preci_type=Single  exp_width=8  frac_width=24  explicit_period=off  period=1  equ=P=C  opselect=C  inp2=PCIN>>17  opr=+  inp1=P  carry=CIN  dbl_ovrd=off  block_type=constant
  Constant12 : xbsIndex_r4/Constant  const=h(13,5)  gui_display_data_type=Fixed-point  arith_type=Signed (2's comp)  n_bits=W  bin_pt=B  preci_type=Single  exp_width=8  frac_width=24  explicit_period=off  period=1  equ=P=C  opselect=C  inp2=PCIN>>17  opr=+  inp1=P  carry=CIN  dbl_ovrd=off  block_type=constant
  Constant13 : xbsIndex_r4/Constant  const=h(14,5)  gui_display_data_type=Fixed-point  arith_type=Signed (2's comp)  n_bits=W  bin_pt=B  preci_type=Single  exp_width=8  frac_width=24  explicit_period=off  period=1  equ=P=C  opselect=C  inp2=PCIN>>17  opr=+  inp1=P  carry=CIN  dbl_ovrd=off  block_type=constant
  Constant14 : xbsIndex_r4/Constant  const=h(15,5)  gui_display_data_type=Fixed-point  arith_type=Signed (2's comp)  n_bits=W  bin_pt=B  preci_type=Single  exp_width=8  frac_width=24  explicit_period=off  period=1  equ=P=C  opselect=C  inp2=PCIN>>17  opr=+  inp1=P  carry=CIN  dbl_ovrd=off  block_type=constant
  Constant15 : xbsIndex_r4/Constant  const=h(16,5)  gui_display_data_type=Fixed-point  arith_type=Signed (2's comp)  n_bits=W  bin_pt=B  preci_type=Single  exp_width=8  frac_width=24  explicit_period=off  period=1  equ=P=C  opselect=C  inp2=PCIN>>17  opr=+  inp1=P  carry=CIN  dbl_ovrd=off  block_type=constant
  Constant16 : xbsIndex_r4/Constant  const=h(17,5)  gui_display_data_type=Fixed-point  arith_type=Signed (2's comp)  n_bits=W  bin_pt=B  preci_type=Single  exp_width=8  frac_width=24  explicit_period=off  period=1  equ=P=C  opselect=C  inp2=PCIN>>17  opr=+  inp1=P  carry=CIN  dbl_ovrd=off  block_type=constant
  Constant2 : xbsIndex_r4/Constant  const=h(3,5)  gui_display_data_type=Fixed-point  arith_type=Signed (2's comp)  n_bits=W  bin_pt=B  preci_type=Single  exp_width=8  frac_width=24  explicit_period=off  period=1  equ=P=C  opselect=C  inp2=PCIN>>17  opr=+  inp1=P  carry=CIN  dbl_ovrd=off  block_type=constant
  Constant3 : xbsIndex_r4/Constant  const=h(4,5)  gui_display_data_type=Fixed-point  arith_type=Signed (2's comp)  n_bits=W  bin_pt=B  preci_type=Single  exp_width=8  frac_width=24  explicit_period=off  period=1  equ=P=C  opselect=C  inp2=PCIN>>17  opr=+  inp1=P  carry=CIN  dbl_ovrd=off  block_type=constant
  Constant4 : xbsIndex_r4/Constant  const=h(5,5)  gui_display_data_type=Fixed-point  arith_type=Signed (2's comp)  n_bits=W  bin_pt=B  preci_type=Single  exp_width=8  frac_width=24  explicit_period=off  period=1  equ=P=C  opselect=C  inp2=PCIN>>17  opr=+  inp1=P  carry=CIN  dbl_ovrd=off  block_type=constant
  Constant5 : xbsIndex_r4/Constant  const=h(6,5)  gui_display_data_type=Fixed-point  arith_type=Signed (2's comp)  n_bits=W  bin_pt=B  preci_type=Single  exp_width=8  frac_width=24  explicit_period=off  period=1  equ=P=C  opselect=C  inp2=PCIN>>17  opr=+  inp1=P  carry=CIN  dbl_ovrd=off  block_type=constant
  Constant6 : xbsIndex_r4/Constant  const=h(7,5)  gui_display_data_type=Fixed-point  arith_type=Signed (2's comp)  n_bits=W  bin_pt=B  preci_type=Single  exp_width=8  frac_width=24  explicit_period=off  period=1  equ=P=C  opselect=C  inp2=PCIN>>17  opr=+  inp1=P  carry=CIN  dbl_ovrd=off  block_type=constant
  Constant7 : xbsIndex_r4/Constant  const=h(8,5)  gui_display_data_type=Fixed-point  arith_type=Signed (2's comp)  n_bits=W  bin_pt=B  preci_type=Single  exp_width=8  frac_width=24  explicit_period=off  period=1  equ=P=C  opselect=C  inp2=PCIN>>17  opr=+  inp1=P  carry=CIN  dbl_ovrd=off  block_type=constant
  Constant8 : xbsIndex_r4/Constant  const=h(9,5)  gui_display_data_type=Fixed-point  arith_type=Signed (2's comp)  n_bits=W  bin_pt=B  preci_type=Single  exp_width=8  frac_width=24  explicit_period=off  period=1  equ=P=C  opselect=C  inp2=PCIN>>17  opr=+  inp1=P  carry=CIN  dbl_ovrd=off  block_type=constant
  Constant9 : xbsIndex_r4/Constant  const=h(10,5)  gui_display_data_type=Fixed-point  arith_type=Signed (2's comp)  n_bits=W  bin_pt=B  preci_type=Single  exp_width=8  frac_width=24  explicit_period=off  period=1  equ=P=C  opselect=C  inp2=PCIN>>17  opr=+  inp1=P  carry=CIN  dbl_ovrd=off  block_type=constant
  Delay{2..17} (16 alike) : xbsIndex_r4/Delay  rst=off  infoeditControl=Selection of Reset will increase slice count due to use of real FFs and instead of SRLs  en=off  latency=1  reg_retiming=off  dbl_ovrd=off  block_type=delay
  Gateway In : xbsIndex_r4/Gateway In  gui_display_data_type=Fixed-point  arith_type="Signed  (2's comp)"  n_bits=W  bin_pt=B  preci_type=Single  exp_width=8  frac_width=24  rows=1  columns=1  quantization="Round  (unbiased: +/- Inf)"  overflow=Saturate  period=st  UseAsADC=off  ADCChannel='1'  interface=None  automatic_assignment=on  address_offset=hex2dec('00')  intf_name=''  intf_description=''  default_value=0  timing_constraint=None  locs_specified=off  LOCs={}  io_standard={}  inherit_from_input=off  hdl_port=on  dbl_ovrd=off  block_type=gatewayin
  Mult{,15..30} (17 alike) : xbsIndex_r4/Mult  precision=User Defined  arith_type="Signed  (2's comp)"  n_bits=W  bin_pt=B  quantization="Round  (unbiased: +/- Inf)"  overflow=Flag as error  en=off  latency=0  use_behavioral_HDL=off  opt=Speed  use_embedded=on  optimum_pipeline=off  pipeline=on  dbl_ovrd=off  use_rpm=on  placement_style=Triangular  block_type=mult
  Out1 : Outport
  wires:
  AddSub2/1 -> Out1/1
  Constant14/1 -> Mult16/2
  Mult/1 -> AddSub16/2
  Mult16/1 -> AddSub1/2
  AddSub16/1 -> Delay15/1
  Constant15/1 -> Mult/2
  AddSub1/1 -> Delay2/1
  Constant13/1 -> Mult17/2
  Mult17/1 -> AddSub18/2
  Constant12/1 -> Mult18/2
  AddSub17/1 -> Delay4/1
  AddSub18/1 -> Delay3/1
  Constant11/1 -> Mult19/2
  Mult19/1 -> AddSub20/2
  Constant10/1 -> Mult20/2
  Mult20/1 -> AddSub19/2
  AddSub19/1 -> Delay6/1
  AddSub20/1 -> Delay5/1
  Constant9/1 -> Mult21/2
  Mult21/1 -> AddSub22/2
  Constant8/1 -> Mult22/2
  AddSub21/1 -> Delay8/1
  AddSub22/1 -> Delay7/1
  Constant7/1 -> Mult23/2
  Mult23/1 -> AddSub24/2
  Constant6/1 -> Mult24/2
  AddSub23/1 -> Delay10/1
  Constant5/1 -> Mult25/2
  Mult25/1 -> AddSub26/2
  Constant4/1 -> Mult26/2
  Mult26/1 -> AddSub25/2
  AddSub25/1 -> Delay12/1
  AddSub26/1 -> Delay11/1
  Constant3/1 -> Mult27/2
  Mult27/1 -> AddSub28/2
  Constant2/1 -> Mult28/2
  AddSub27/1 -> Delay14/1
  AddSub28/1 -> Delay13/1
  Constant1/1 -> Mult29/2
  Mult29/1 -> AddSub30/2
  Constant/1 -> Mult30/2
  Mult30/1 -> Delay17/1
  AddSub30/1 -> Delay16/1
  AddSub24/1 -> Delay9/1
  Delay2/1 -> AddSub16/1
  Delay3/1 -> AddSub1/1
  Delay4/1 -> AddSub18/1
  Delay6/1 -> AddSub20/1
  Delay7/1 -> AddSub19/1
  Delay8/1 -> AddSub22/1
  Delay10/1 -> AddSub24/1
  Delay12/1 -> AddSub26/1
  Delay13/1 -> AddSub25/1
  Delay14/1 -> AddSub28/1
  Delay17/1 -> AddSub30/1
  Constant16/1 -> Mult15/2
  Mult15/1 -> AddSub2/2
  Delay15/1 -> AddSub2/1
  In1/1 -> Gateway In/1
  Delay5/1 -> AddSub17/1
  Mult18/1 -> AddSub17/2
  Delay9/1 -> AddSub21/1
  Mult22/1 -> AddSub21/2
  Delay11/1 -> AddSub23/1
  Mult24/1 -> AddSub23/2
  Delay16/1 -> AddSub27/1
  Mult28/1 -> AddSub27/2
  Gateway In/1 -> Mult30/1, Mult29/1, Mult28/1, Mult27/1, Mult26/1, Mult25/1, Mult24/1, Mult22/1, Mult21/1, Mult19/1, Mult17/1, Mult15/1, Mult/1, Mult16/1, Mult18/1, Mult20/1, Mult23/1
